simulink model "SignalModelL5"  (R2017a)
settings: Solver=FixedStepAuto  StartTime=0.0  StopTime=10  FixedStep=0.01  RelTol=1e-3
undefined symbols (not defined in the file): a, A2, b2, u2
settings Model: Creator=roman  LastModifiedBy=roman

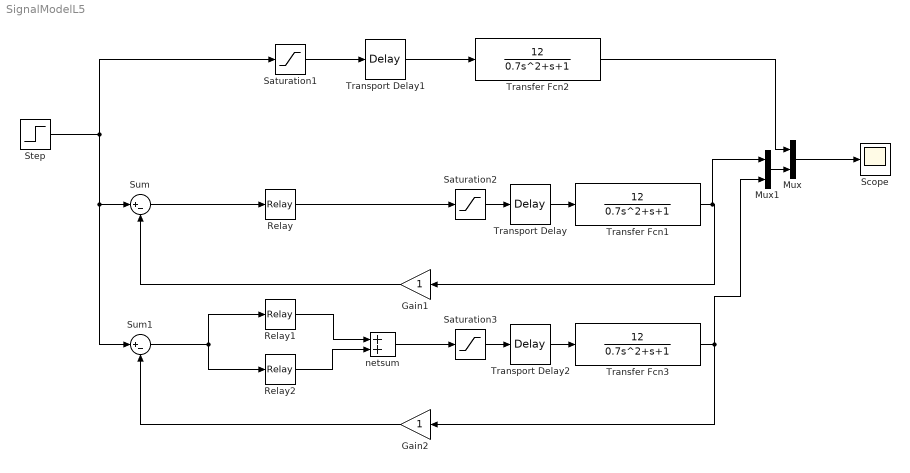
== system SignalModelL5 ==
  Gain1 : Gain
  Gain2 : Gain
  Mux : Mux  Inputs=2
  Mux1 : Mux  Inputs=2
  Relay : Relay  OnSwitchValue=a  OffSwitchValue=-a  OnOutputValue=u  OffOutputValue=-u
  Relay1 : Relay  OnSwitchValue=u2+b2  OffSwitchValue=u2  OnOutputValue=A2
  Relay2 : Relay  OnSwitchValue=-u2  OffSwitchValue=-u2-b2  OnOutputValue=0  OffOutputValue=-A2
  Saturation1 : Saturate  UpperLimit=2000  LowerLimit=-2000
  Saturation2 : Saturate  UpperLimit=2000  LowerLimit=-2000
  Saturation3 : Saturate  UpperLimit=2000  LowerLimit=-2000
  Scope : Scope
  Step : Step  Time=0  SampleTime=0
  Sum : Sum  Inputs=|+-
  Sum1 : Sum  Inputs=|+-
  Transfer Fcn1 : TransferFcn  Numerator=[12]  Denominator=[0.7 1 1]
  Transfer Fcn2 : TransferFcn  Numerator=[12]  Denominator=[0.7 1 1]
  Transfer Fcn3 : TransferFcn  Numerator=[12]  Denominator=[0.7 1 1]
  Transport Delay : TransportDelay  DelayTime=0.1
  Transport Delay1 : TransportDelay  DelayTime=0.1
  Transport Delay2 : TransportDelay  DelayTime=0.1
  netsum : Sum  Inputs=2  SaturateOnIntegerOverflow=on  InputSameDT=on  OutDataTypeStr=Inherit: Same as first input
  wires:
  Transport Delay/1 -> Transfer Fcn1/1
  Transfer Fcn1/1 -> Mux1/1, Gain1/1
  Transport Delay1/1 -> Transfer Fcn2/1
  Mux/1 -> Scope/1
  Saturation2/1 -> Transport Delay/1
  Gain1/1 -> Sum/2
  Saturation1/1 -> Transport Delay1/1
  Relay/1 -> Saturation2/1
  Sum/1 -> Relay/1
  Transfer Fcn3/1 -> Mux1/2, Gain2/1
  Saturation3/1 -> Transport Delay2/1
  Step/1 -> Saturation1/1, Sum1/1, Sum/1
  Transport Delay2/1 -> Transfer Fcn3/1
  Relay1/1 -> netsum/1
  Relay2/1 -> netsum/2
  netsum/1 -> Saturation3/1
  Gain2/1 -> Sum1/2
  Mux1/1 -> Mux/2
  Sum1/1 -> Relay2/1, Relay1/1
  Transfer Fcn2/1 -> Mux/1
